simulink model "HPS_5130_Maschinensatz"  (R2022b)
settings: Solver=VariableStepAuto  StartTime=0.0  StopTime=2  RelTol=1e-3
model workspace (MAT data in the model file):
  D_0 = Simulink.Parameter
  D_0.Value = 0.00057
  D_0.Description = 'Reibung konstant
    | '
  D_0.DataType = 'auto'
  D_0.Min = 0
  D_0.Max = 100
  D_0.DocUnits = '(N*m)'
  D_0.Complexity = 'real'
  D_0.Dimensions = [1 1]
  D_R = Simulink.Parameter
  D_R.Value = 9.9e-06
  D_R.Description = 'Konstante für Reibungsmoment'
  D_R.DataType = 'auto'
  D_R.Min = 0
  D_R.Max = 1000
  D_R.DocUnits = 'N*m/rad/sec'
  D_R.Complexity = 'real'
  D_R.Dimensions = [1 1]
  J = Simulink.Parameter
  J.Value = 6.34e-06
  J.Description = 'Trägheitsmoment gesamter Aufbau'
  J.DataType = 'auto'
  J.Min = 0
  J.Max = 200
  J.DocUnits = 'N*m/rad/(sec*sec)'
  J.Complexity = 'real'
  J.Dimensions = [1 1]
  J_S = Simulink.Parameter
  J_S.Value = 1.9e-05
  J_S.Description = 'Gesamtträgheit mit elektrischer Schwungmasse
    | '
  J_S.DataType = 'auto'
  J_S.Complexity = 'real'
  J_S.Dimensions = [1 1]
  K_M = Simulink.Parameter
  K_M.Value = 0.0148
  K_M.Description = 'Drehmomentkonstante
    | '
  K_M.DataType = 'auto'
  K_M.Min = 0
  K_M.Max = 100
  K_M.DocUnits = '(N*m)/A'
  K_M.Complexity = 'real'
  K_M.Dimensions = [1 1]
  K_N = Simulink.Parameter
  K_N.Value = 11.78
  K_N.Description = 'Drehzahlkonstante, 1/Generatorkonstante'
  K_N.DataType = 'auto'
  K_N.Min = 0
  K_N.Max = 1000
  K_N.DocUnits = 'rad/sec/V'
  K_N.Complexity = 'real'
  K_N.Dimensions = [1 1]
  L_A = Simulink.Parameter
  L_A.Value = 0.001
  L_A.Description = 'Wiklungsinduktivität Anker
    | '
  L_A.DataType = 'auto'
  L_A.Min = 0
  L_A.Max = 1
  L_A.DocUnits = 'H'
  L_A.Complexity = 'real'
  L_A.Dimensions = [1 1]
  R_A = Simulink.Parameter
  R_A.Value = 11.9
  R_A.Description = 'Ankerwiderstand
    | 
    | 
    | '
  R_A.DataType = 'auto'
  R_A.Min = 0
  R_A.Max = 200
  R_A.DocUnits = 'Ohm'
  R_A.Complexity = 'real'
  R_A.Dimensions = [1 1]
  R_L = Simulink.Parameter
  R_L.Value = 33
  R_L.Description = 'Strommesswiderstand
    | '
  R_L.DataType = 'auto'
  R_L.Min = 0
  R_L.Max = 100
  R_L.DocUnits = 'Ohm'
  R_L.Complexity = 'real'
  R_L.Dimensions = [1 1]
  R_M = Simulink.Parameter
  R_M.Value = 1
  R_M.Description = 'Strommesswiderstand
    | '
  R_M.DataType = 'auto'
  R_M.Min = 0
  R_M.Max = 10
  R_M.DocUnits = 'Ohm'
  R_M.Complexity = 'real'
  R_M.Dimensions = [1 1]
settings Model: Creator=mathi  LastModifiedBy=mathi

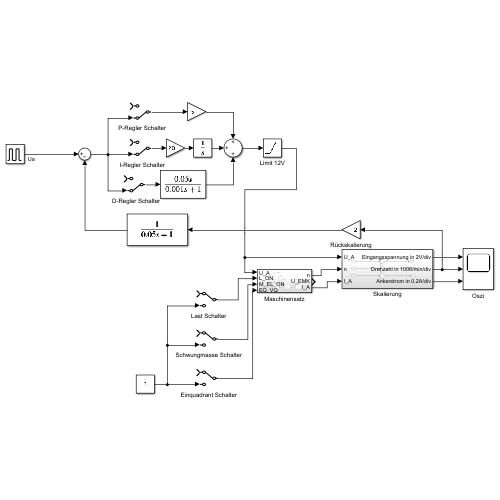
[thumbnail: Simulink's stored preview of the top-level diagram]
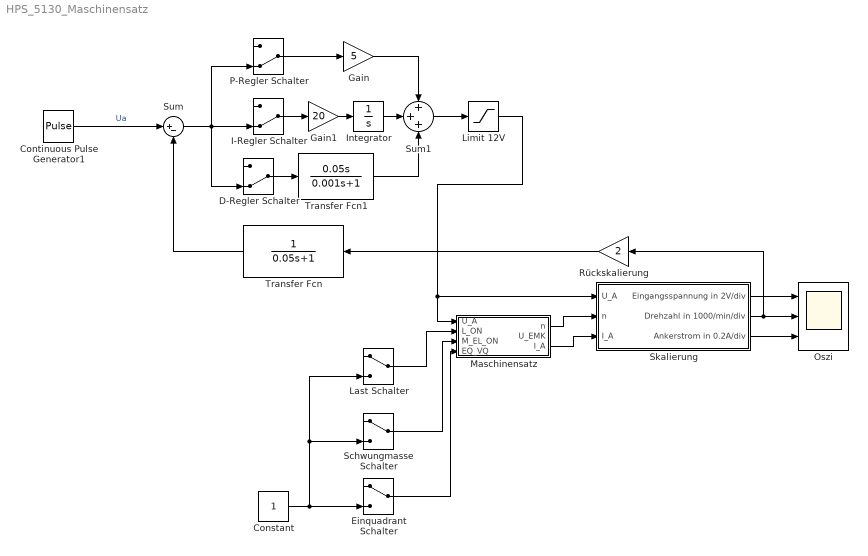
== system HPS_5130_Maschinensatz ==
  Constant : Constant
  Continuous Pulse Generator1 : DiscretePulseGenerator  PulseType=Time based  Amplitude=8  Period=4  PulseWidth=25  PhaseDelay=0.1
  D-Regler Schalter : ManualSwitch  CurrentSetting=0
  Einquadrant Schalter : ManualSwitch
  Gain : Gain  Gain=5
  Gain1 : Gain  Gain=20
  I-Regler Schalter : ManualSwitch  CurrentSetting=0
  Integrator : Integrator
  Last Schalter : ManualSwitch
  Limit 12V : Saturate  UpperLimit=12  LowerLimit=0
  Maschinensatz : Subsystem
  Oszi : Scope  NumInputPorts=3
  P-Regler Schalter : ManualSwitch  CurrentSetting=0
  Rückskalierung : Gain  Gain=2
  Schwungmasse Schalter : ManualSwitch
  Skalierung : Subsystem
  Sum : Sum  Inputs=|+-
  Sum1 : Sum  Inputs=+++
  Transfer Fcn : TransferFcn  Denominator=[0.05 1]
  Transfer Fcn1 : TransferFcn  Numerator=[0.05 0]  Denominator=[0.001 1]
  wires:
  Last Schalter/1 -> Maschinensatz/2(L_ON)
  Constant/1 -> Einquadrant Schalter/2, Schwungmasse Schalter/2, Last Schalter/2
  Schwungmasse Schalter/1 -> Maschinensatz/3(M_EL_ON)
  Maschinensatz/1(n) -> Skalierung/2(n)
  Maschinensatz/3(I_A) -> Skalierung/3(I_A)
  Skalierung/1(Eingangsspannung in 2V/div) -> Oszi/1
  Skalierung/2(Drehzahl in 1000/min/div) -> Rückskalierung/1, Oszi/2
  Skalierung/3(Ankerstrom in 0.2A/div) -> Oszi/3
  Einquadrant Schalter/1 -> Maschinensatz/4(EQ_VQ)
  Sum/1 -> D-Regler Schalter/2, P-Regler Schalter/2, I-Regler Schalter/2
  Transfer Fcn/1 -> Sum/2
  Integrator/1 -> Sum1/2
  Gain1/1 -> Integrator/1
  Gain/1 -> Sum1/1
  Rückskalierung/1 -> Transfer Fcn/1
  Continuous Pulse Generator1/1 -> Sum/1  "Ua"
  Transfer Fcn1/1 -> Sum1/3
  P-Regler Schalter/1 -> Gain/1
  I-Regler Schalter/1 -> Gain1/1
  Limit 12V/1 -> Skalierung/1(U_A), Maschinensatz/1(U_A)
  D-Regler Schalter/1 -> Transfer Fcn1/1
  Sum1/1 -> Limit 12V/1

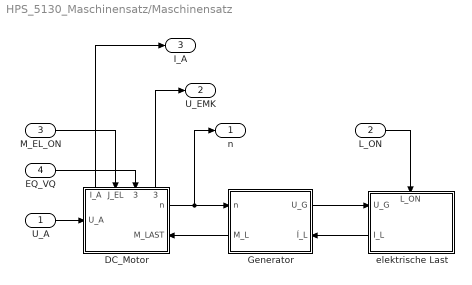
== system HPS_5130_Maschinensatz/Maschinensatz ==
  U_A : Inport
  L_ON : Inport  Port=2
  M_EL_ON : Inport  Port=3
  EQ_VQ : Inport  Port=4
  DC_Motor : Subsystem
      settings: PortSchema="{\"entries\":[{\"content\":{\"sides\":[{\"content\":{\"connectorIds\":[\"In1\"]},\"type\":\"ConnectorPlacement.EquallySpacedRectSide\",\"uuid\":\"35393a06-0abc-425e-a196-e2b70b805d15\"},{\"content\":{\"connectorIds\":[\"Out1\",\"In4\"],\"side\":\"RIGHT\"},\"type\":\"ConnectorPlacement.EquallySpacedRectSide\",\"uuid\":\"36638641-2bf7-4234-945e-525f833f6a48\"},{\"content\":{\"connectorIds\":[\"Out2\",\"In2\",\"In3\",\"Out3\"],\"side\":\"TOP\"},\"type\":\"ConnectorPlacement.EquallySpacedRectSide\",\"uuid\":\"2bb2e75b-dd4a-4523-bd4d-6af904bc993e\"}]},\"type\":\"ConnectorPlacement.EquallySpacedConnector\",\"uuid\":\"b93f7a08-ff8a-4269-8405-af0864ace3db\"}],\"packageUris\":[\"http://schema.mathworks.com/mf0/Connector/R2020b\"],\"version\":\"1.0\"}"
  Generator : Subsystem
      settings: PortSchema="{\"entries\":[{\"content\":{\"sides\":[{\"content\":{\"connectorIds\":[\"In1\",\"Out2\"]},\"type\":\"ConnectorPlacement.EquallySpacedRectSide\",\"uuid\":\"fae34ad4-846a-4100-8540-e82bea0aa29d\"},{\"content\":{\"connectorIds\":[\"Out1\",\"In2\"],\"side\":\"RIGHT\"},\"type\":\"ConnectorPlacement.EquallySpacedRectSide\",\"uuid\":\"26f3a1e3-dc9c-4d6a-b60a-b904a0098d1f\"},{\"content\":{\"connectorIds\":[],\"side\":\"TOP\"},\"type\":\"ConnectorPlacement.EquallySpacedRectSide\",\"uuid\":\"09074506-074c-47d5-bd87-fa0f9f7b8901\"}]},\"type\":\"ConnectorPlacement.EquallySpacedConnector\",\"uuid\":\"8b2f8229-34e5-4770-bf5a-e25e1bd29f7d\"}],\"packageUris\":[\"http://schema.mathworks.com/mf0/Connector/R2020b\"],\"version\":\"1.0\"}"
  elektrische Last : Subsystem
      settings: PortSchema="{\"entries\":[{\"content\":{\"sides\":[{\"content\":{\"connectorIds\":[\"In1\",\"Out1\"]},\"type\":\"ConnectorPlacement.EquallySpacedRectSide\",\"uuid\":\"4cad360b-76b6-44be-9fdf-f7be0d2e4a17\"},{\"content\":{\"connectorIds\":[],\"side\":\"RIGHT\"},\"type\":\"ConnectorPlacement.EquallySpacedRectSide\",\"uuid\":\"3d37b72b-42e7-438c-bc29-4e42c6d66069\"},{\"content\":{\"connectorIds\":[\"In2\"],\"side\":\"TOP\"},\"type\":\"ConnectorPlacement.EquallySpacedRectSide\",\"uuid\":\"b5d7fa8c-707a-43b8-94be-94db05fe57fe\"}]},\"type\":\"ConnectorPlacement.EquallySpacedConnector\",\"uuid\":\"4d74878e-f26c-456a-9066-a676593611b8\"}],\"packageUris\":[\"http://schema.mathworks.com/mf0/Connector/R2020b\"],\"version\":\"1.0\"}"
  n : Outport
  U_EMK : Outport  Port=2
  I_A : Outport  Port=3
  wires:
  U_A/1 -> DC_Motor/1(U_A)
  DC_Motor/1(n) -> n/1, Generator/1(n)
  DC_Motor/2(I_A) -> I_A/1
  L_ON/1 -> elektrische Last/2(L_ON)
  Generator/1(U_G) -> elektrische Last/1(U_G)
  elektrische Last/1(I_L) -> Generator/2(Í_L)
  Generator/2(M_L) -> DC_Motor/4(M_LAST)
  M_EL_ON/1 -> DC_Motor/2(J_EL)
  EQ_VQ/1 -> DC_Motor/3(EQ_VQ)
  DC_Motor/3(U_EMK) -> U_EMK/1

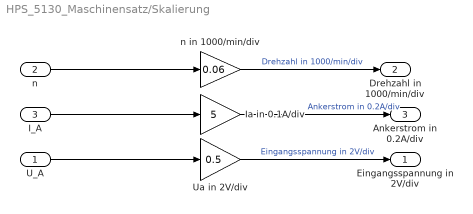
== system HPS_5130_Maschinensatz/Skalierung ==
  U_A : Inport
  n : Inport  Port=2
  I_A : Inport  Port=3
  Ia in 0.1A/div : Gain  Gain=5
  Ua in 2V/div : Gain  Gain=0.5
  n in 1000/min/div : Gain  Gain=0.06
  Eingangsspannung in 2V/div : Outport
  Drehzahl in 1000/min/div : Outport  Port=2
  Ankerstrom in 0.2A/div : Outport  Port=3
  wires:
  Ua in 2V/div/1 -> Eingangsspannung in 2V/div/1  "Eingangsspannung in 2V/div"
  n in 1000/min/div/1 -> Drehzahl in 1000/min/div/1  "Drehzahl in 1000/min/div"
  U_A/1 -> Ua in 2V/div/1
  n/1 -> n in 1000/min/div/1
  I_A/1 -> Ia in 0.1A/div/1
  Ia in 0.1A/div/1 -> Ankerstrom in 0.2A/div/1  "Ankerstrom in 0.2A/div"

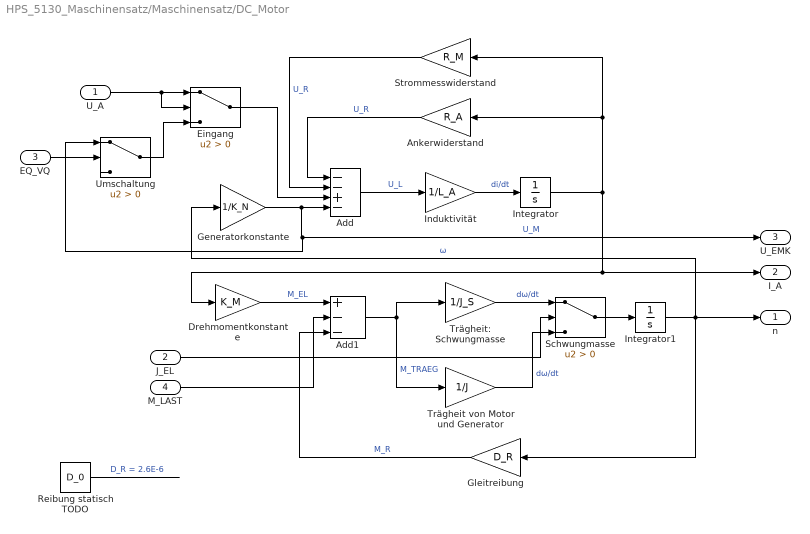
== system HPS_5130_Maschinensatz/Maschinensatz/DC_Motor ==
  U_A : Inport
  J_EL : Inport  Port=2
  EQ_VQ : Inport  Port=3
  M_LAST : Inport  Port=4
  Add : Sum  Inputs=--+-
  Add1 : Sum  Inputs=+--
  Ankerwiderstand : Gain  Gain=R_A
  Drehmomentkonstante : Gain  Gain=K_M
  Eingang : Switch  Criteria=u2 > Threshold  SaturateOnIntegerOverflow=off  InputSameDT=off
  Generatorkonstante : Gain  Gain=1/K_N
  Gleitreibung : Gain  Gain=D_R
  Induktivität : Gain  Gain=1/L_A
  Integrator : Integrator
  Integrator1 : Integrator
  Reibung statisch TODO : Constant  Value=D_0
  Schwungmasse : Switch  Criteria=u2 > Threshold  SaturateOnIntegerOverflow=off  InputSameDT=off
  Strommesswiderstand : Gain  Gain=R_M
  Trägheit von Motor und Generator : Gain  Gain=1/J
  Trägheit: Schwungmasse : Gain  Gain=1/J_S
  Umschaltung : Switch  Criteria=u2 > Threshold  SaturateOnIntegerOverflow=off  InputSameDT=off
  n : Outport
  I_A : Outport  Port=2
  U_EMK : Outport  Port=3
  wires:
  Induktivität/1 -> Integrator/1  "di/dt"
  Integrator/1 -> I_A/1, Drehmomentkonstante/1, Ankerwiderstand/1, Strommesswiderstand/1
  Ankerwiderstand/1 -> Add/1  "U_R"
  Add/1 -> Induktivität/1  "U_L"
  Generatorkonstante/1 -> Umschaltung/1, U_EMK/1, Add/4  "U_M"
  Strommesswiderstand/1 -> Add/2  "U_R"
  Drehmomentkonstante/1 -> Add1/1  "M_EL"
  Integrator1/1 -> Gleitreibung/1, Generatorkonstante/1, n/1  "ω"
  Reibung statisch TODO/1 -> ?  "D_R = 2.6E-6"
  Add1/1 -> Trägheit von Motor und Generator/1, Trägheit: Schwungmasse/1  "M_TRAEG"
  Trägheit: Schwungmasse/1 -> Schwungmasse/1  "dω/dt"
  Schwungmasse/1 -> Integrator1/1
  Trägheit von Motor und Generator/1 -> Schwungmasse/3  "dω/dt"
  J_EL/1 -> Schwungmasse/2
  U_A/1 -> Eingang/2, Eingang/1
  Eingang/1 -> Add/3
  Umschaltung/1 -> Eingang/3
  EQ_VQ/1 -> Umschaltung/2
  M_LAST/1 -> Add1/2
  Gleitreibung/1 -> Add1/3  "M_R"

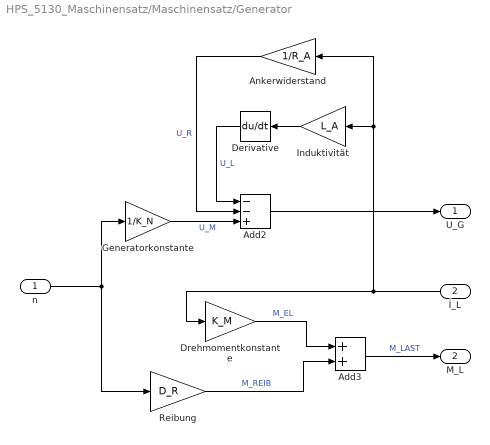
== system HPS_5130_Maschinensatz/Maschinensatz/Generator ==
  n : Inport
  Í_L : Inport  Port=2
  Add2 : Sum  Inputs=--+
  Add3 : Sum
  Ankerwiderstand : Gain  Gain=1/R_A
  Derivative : Derivative
  Drehmomentkonstante : Gain  Gain=K_M
  Generatorkonstante : Gain  Gain=1/K_N
  Induktivität : Gain  Gain=L_A
  Reibung : Gain  Gain=D_R
  U_G : Outport
  M_L : Outport  Port=2
  wires:
  Í_L/1 -> Ankerwiderstand/1, Induktivität/1, Drehmomentkonstante/1
  Ankerwiderstand/1 -> Add2/2  "U_R"
  n/1 -> Reibung/1, Generatorkonstante/1
  Induktivität/1 -> Derivative/1
  Derivative/1 -> Add2/1  "U_L"
  Generatorkonstante/1 -> Add2/3  "U_M"
  Add2/1 -> U_G/1
  Reibung/1 -> Add3/2  "M_REIB"
  Drehmomentkonstante/1 -> Add3/1  "M_EL"
  Add3/1 -> M_L/1  "M_LAST"

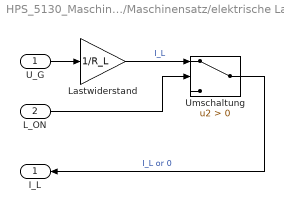
== system HPS_5130_Maschinensatz/Maschinensatz/elektrische Last ==
  U_G : Inport
  L_ON : Inport  Port=2
  Lastwiderstand : Gain  Gain=1/R_L
  Umschaltung : Switch  Criteria=u2 > Threshold  SaturateOnIntegerOverflow=off  InputSameDT=off
  I_L : Outport
  wires:
  L_ON/1 -> Umschaltung/2
  Lastwiderstand/1 -> Umschaltung/1  "I_L"
  Umschaltung/1 -> I_L/1  "I_L or 0"
  U_G/1 -> Lastwiderstand/1
